simulink model "hdlFrame_RGBFilter_MLFB"  (R2023a)
settings: Solver=FixedStepDiscrete  StartTime=0.0  StopTime=2  RelTol=1e-3
InitFcn:
  | R = 752;
  | C = 480;
  | redMax = 0;
  | greenMax = 255;
  | blueMax = 0;
undefined symbols (not defined in the file or in its folder): gray
libraries: visionsources x1
Description:
  | Sobel Edge Detection Using the MATLAB(R) Function Block
  | This example shows how to use HDL Coder(TM) to check,
  | generate, and verify HDL code for a Sobel Edge Detection
  | block built using the MATLAB Function block.
settings Model: Creator=The MathWorks, Inc.  LastModifiedBy=navan
settings SolverCC: AlgebraicLoopSolver=TrustRegion  MaxZcPerStep=1
settings DataIOCC: LimitDataPoints=on  SaveFormat=Array  SignalLogging=off  ReturnWorkspaceOutputs=off
settings OptimizationCC: BlockReduction=off  ConditionallyExecuteInputs=off  DefaultParameterBehavior=Inlined  ReuseModelBlockBuffer=off  ExpressionDepthLimit=2147483647  InitFltsAndDblsToZero=on  EfficientMapNaN2IntZero=off  LifeSpan=inf
settings DebuggingCC: AlgebraicLoopMsg=error  SaveWithParameterizedLinksMsg=none  UnderspecifiedInitializationDetection=Classic  MergeDetectMultiDrivingBlocksExec=none  SignalResolutionControl=TryResolveAllWithWarning  MultiTaskDSMMsg=warning  MultiTaskCondExecSysMsg=none  SingleTaskRateTransMsg=error  IntegerOverflowMsg=none  ParameterPrecisionLossMsg=none  FcnCallInpInsideContextMsg=warning  UnconnectedInputMsg=warning  UnconnectedOutputMsg=warning  UnconnectedLineMsg=warning  AllowSymbolicDim=off  StateNameClashWarn=warning  StrictBusMsg=ErrorOnBusTreatedAsVector  SFUnexpectedBacktrackingDiag=warning  SFNoUnconditionalDefaultTransitionDiag=warning  SFExecutionAtInitializationDiag=none  IntegerSaturationMsg=none  ArithmeticOperatorsInVariantConditions=warning
settings HardwareCC: ProdBitPerPointer=32  ProdBitPerSizeT=32  ProdBitPerPtrDiffT=32  ProdLargestAtomicFloat=None  ProdIntDivRoundTo=Undefined  ProdEndianess=Unspecified  ProdWordSize=32  ProdHWDeviceType=ASIC/FPGA  TargetHWDeviceType=32-bit Generic  ProdEqTarget=off
settings ModelReferenceCC: EnableRefExpFcnMdlSchedulingChecks=on  PropagateSignalLabelsOutOfModel=off
settings SFSimCC: SimUseLocalCustomCode=off  CustomCodeUndefinedFunction=UseInterfaceOnly
settings RTWCC: RTWUseLocalCustomCode=off  DLArmComputeVersion=19.05
settings CodeAppCC: StateflowObjectComments=on
settings GRTTargetCC: TargetFcnLib=ansi_tfl_tmw.mat  TargetLangStandard=C89/C90 (ANSI)  CombineOutputUpdateFcns=off  GRTInterface=on
settings ConfigComp: CovMetricSettings=dw  CovSaveCumulativeToWorkspaceVar=on  CovSaveSingleToWorkspaceVar=on  CovExternalEMLEnable=off

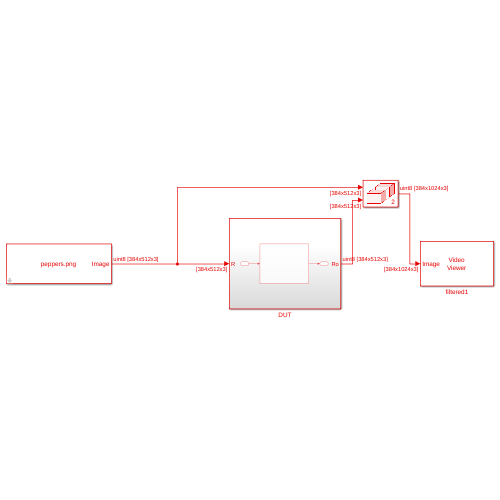
[thumbnail: Simulink's stored preview of the top-level diagram]
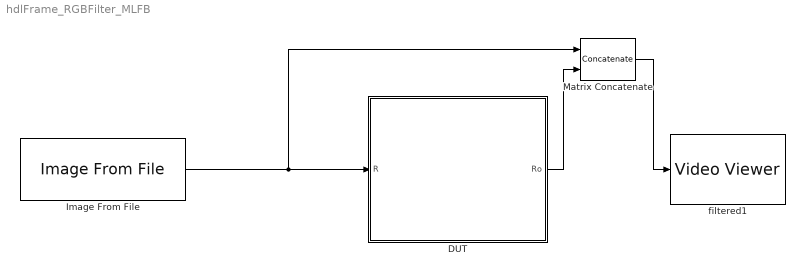
== system hdlFrame_RGBFilter_MLFB ==
  DUT : Subsystem
  Image From File : visionsources/Image From File  Tag=vipblks_nd  FileName=peppers.png  Ts=1  imagePorts=One multidimensional signal  OutPortLabels=R|G|B  ImageDataType=Inherit from input image  sdImageDataType=uint(8)  Signed=on  WordLength=16  FractionLengthMode=User-defined  FractionLength=15
  Matrix Concatenate : Concatenate  Mode=Multidimensional array  ConcatenateDimension=2
  filtered1 : VideoViewer  colormapValue=gray(256)  FigPos=[227.666666666667 1280 1280 622.666666666667]
  wires:
  DUT/1(Ro) -> Matrix Concatenate/2
  Image From File/1 -> Matrix Concatenate/1, DUT/1(R)
  Matrix Concatenate/1 -> filtered1/1

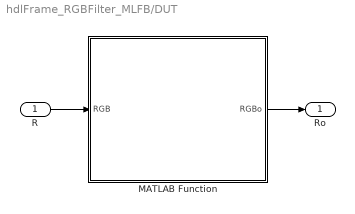
== system hdlFrame_RGBFilter_MLFB/DUT ==
  R : Inport
  MATLAB Function : MATLAB Function  TreatAsAtomicUnit=on
  Ro : Outport
  wires:
  MATLAB Function/1(RGBo) -> Ro/1
  R/1 -> MATLAB Function/1(RGB)

== matlab function hdlFrame_RGBFilter_MLFB/DUT/MATLAB Function ==
  data: RGB input; RGBo output
function RGBo  = fcn(RGB)


R = RGB(:,:,1);
G = RGB(:,:,2);
B = RGB(:,:,3);

coder.inline('always');

[Ro, Go, Bo] = hdl.npufun(@imfilter_kernel, [1 1], R, G, B);

RGBo = cat(3, Ro, Go, Bo);

end

function [Ro, Go, Bo] = imfilter_kernel(R, G, B)

coder.inline('always');

redMax = uint8(255);
greenMax = uint8(0);
blueMax = uint8(0);

if R <= redMax
    Ro = R;
else
    Ro = uint8(0);
end

if G <= greenMax
    Go = G;
else
    Go = uint8(0);
end
    
if B <= blueMax
    Bo = B;
else
    Bo = uint8(0);
end

end
